simulink model "codegen_01"  (R2013b)
settings: Solver=ode3  StartTime=0.0  StopTime=10.0  RelTol=1e-3
InitFcn:
  | k = 5;
settings Model: BufferReuse=off  Creator=Administrator  LastModifiedBy=Administrator
settings OptimizationCC: InlineParams=on  OptimizeBlockIOStorage=off  BufferReuse=off  ExpressionFolding=off  LocalBlockOutputs=off  OptimizeModelRefInitCode=on  LifeSpan=1
settings HardwareCC: ProdHWDeviceType=Generic->32-bit Embedded Processor
settings RTWCC: SystemTargetFile=ert.tlc  GenCodeOnly=on  TemplateMakefile=ert_default_tmf  Description=Embedded Coder  GenerateReport=on  ProcessScript=ert_make_rtw_hook  IncludeHyperlinkInReport=on  LaunchReport=on
settings CodeAppCC: IgnoreCustomStorageClasses=off  ReqsInCode=on
settings ERTTargetCC: CodeReplacementLibrary=ANSI_C  GenerateSampleERTMain=on  GeneratePreprocessorConditionals=Disable all  CombineSignalStateStructs=on  SuppressErrorStatus=on  ERTCustomFileTemplate=example_file_process.tlc  MemSecPackage=Simulink

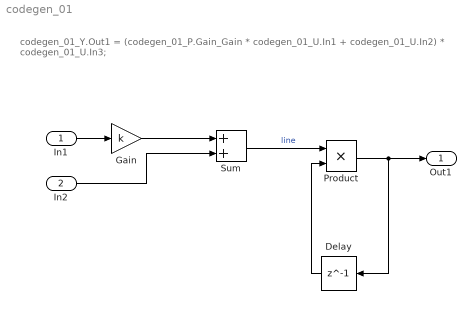
== system codegen_01 ==
  note: codegen_01_Y.Out1 = (codegen_01_P.Gain_Gain * codegen_01_U.In1 +
      |                      codegen_01_U.In2) * codegen_01_U.In3;
  In1 : Inport
  In2 : Inport  Port=2
  Delay : Delay  DelayLength=1  InitialCondition=0
  Gain : Gain  Gain=k
  Product : Product
  Sum : Sum
  Out1 : Outport
  wires:
  In1/1 -> Gain/1
  In2/1 -> Sum/2
  Sum/1 -> Product/1  "line"
  Product/1 -> Delay/1, Out1/1
  Gain/1 -> Sum/1
  Delay/1 -> Product/2
